simulink model "sldemo_lct_work"  (Simulink 7.6)
settings: Solver=ode5  StartTime=0.0  StopTime=1  RelTol=1e-3
PreLoadFcn:
  | load sldemo_lct_data.mat
Description:
  | Structure Arguments Using Buses
settings Model: Creator=The MathWorks Inc.  ExtModeAutoUpdateStatusClock=off
settings DataIOCC: SignalLoggingName=logsOut
settings OptimizationCC: InlineParams=on  InlineInvariantSignals=on  InitFltsAndDblsToZero=on
settings DebuggingCC: CheckExecutionContextPreStartOutputMsg=on  CheckExecutionContextRuntimeOutputMsg=on  SignalResolutionControl=TryResolveAllWithWarning  SolverPrmCheckMsg=none  MultiTaskDSMMsg=warning  MultiTaskCondExecSysMsg=none  BusObjectLabelMismatch=error  StrictBusMsg=ErrorOnBusTreatedAsVector
settings HardwareCC: TargetHWDeviceType=32-bit Generic
settings ModelReferenceCC: UpdateModelReferenceTargets=IfOutOfDate
settings RTWCC: GenerateReport=on  RetainRTWFile=on  ProcessScript=grt_make_rtw_hook  CustomInclude=.\src  LaunchReport=on  IncludeERTFirstTime=on
settings GRTTargetCC: TargetFcnLib=ansi_tfl_tmw.mat

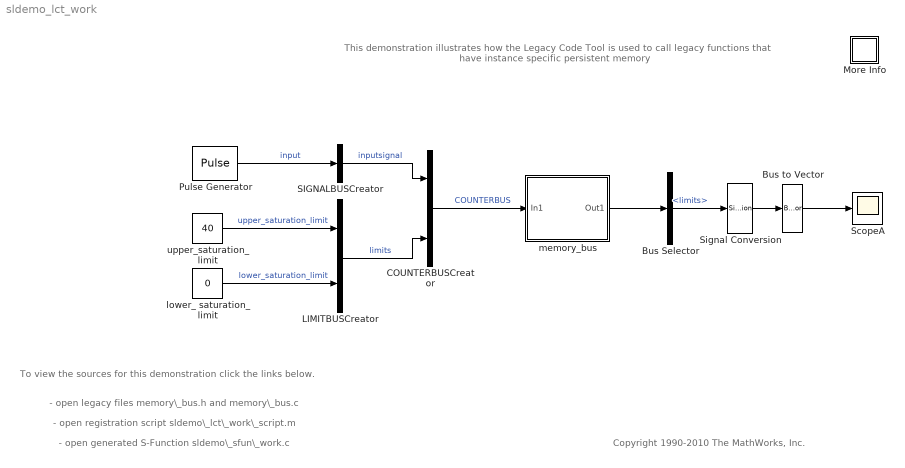
== system sldemo_lct_work ==
  note: This demonstration illustrates how the Legacy Code Tool is used to
      | call legacy functions that have instance specific persistent memory
  note: Copyright 1990-2010 The MathWorks, Inc.
  note: - open legacy files memory\_bus.h and memory\_bus.c
  note: To view the sources for this demonstration
      | click the links below.
  note: - open registration script sldemo\_lct\_work\_script.m
  note: - open generated S-Function sldemo\_sfun\_work.c
  Bus Selector : BusSelector  OutputSignals=limits
  Bus to Vector : BusToVector
  COUNTERBUSCreator : BusCreator  Inputs=2  OutDataTypeStr=Bus: COUNTERBUS  NonVirtualBus=on
  LIMITBUSCreator : BusCreator  Inputs=2  OutDataTypeStr=Bus: LIMITBUS  NonVirtualBus=on
  More Info : Subsystem
      settings: OpenFcn=showdemo('sldemo_lct_work_script')
      mask Display: disp('?')
  Pulse Generator : DiscretePulseGenerator  Amplitude=int32(1)  SampleTime=0.1
  SIGNALBUSCreator : BusCreator  Inputs=1  OutDataTypeStr=Bus: SIGNALBUS  NonVirtualBus=on
  ScopeA : Scope
      settings: TimeRange=1  YMin=-10  YMax=40  SaveName=ScopeDataA  DataFormat=Array
  Signal Conversion : SignalConversion  ConversionOutput=Virtual bus
  lower_ saturation_ limit : Constant  Value=0  OutDataTypeStr=int32
  memory_bus : Subsystem
  upper_saturation_limit : Constant  Value=40  OutDataTypeStr=int32
  wires:
  upper_saturation_limit/1 -> LIMITBUSCreator/1  "upper_saturation_limit"
  lower_ saturation_ limit/1 -> LIMITBUSCreator/2  "lower_saturation_limit"
  LIMITBUSCreator/1 -> COUNTERBUSCreator/2  "limits"
  Pulse Generator/1 -> SIGNALBUSCreator/1  "input"
  SIGNALBUSCreator/1 -> COUNTERBUSCreator/1  "inputsignal"
  memory_bus/1(Out1) -> Bus Selector/1
  COUNTERBUSCreator/1 -> memory_bus/1(In1)  "COUNTERBUS"
  Bus Selector/1 -> Signal Conversion/1  "<limits>"
  Signal Conversion/1 -> Bus to Vector/1
  Bus to Vector/1 -> ScopeA/1

== system sldemo_lct_work/More Info ==

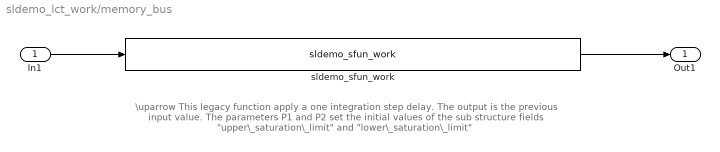
== system sldemo_lct_work/memory_bus ==
  note: \uparrow
      | This legacy function apply a one integration step delay. The output is the previous input value.
      | The parameters P1 and P2 set the initial values of the sub structure fields "upper\_saturation\_limit" and
      | "lower\_saturation\_limit"
  In1 : Inport  OutDataTypeStr=Bus: COUNTERBUS
  sldemo_sfun_work : S-Function  FunctionName=sldemo_sfun_work  Parameters=SParameter1, SParameter2  EnableBusSupport=off  mask(Legacy Function){SFunctionSpec=void memory_bus_step(COUNTERBUS u1[1], COUNTERBUS work1[1], COUNTERBUS y1[1]), SParameter1=10, SParameter2=-10, ShowSpec=on}
      mask prompts: SParameter1 "P1:"; SParameter2 "P2:"; ShowSpec "Display function specification"
      mask help:
      | This block allows you to call the legacy functions specified by the following Legacy Code Tool definition:
      | def.SFunctionName = 'sldemo_sfun_work';
      | def.InitializeConditionsFcnSpec = 'void memory_bus_init(COUNTERBUS work1[1], int32 p1, int32 p2)';
      | def.OutputFcnSpec = 'void memory_bus_step(COUNTERBUS u1[1], COUNTERBUS work1[1], COUNTERBUS y1[1])';
      | def.HeaderFiles = {'memory_bus.h'};
      | def.SourceFiles = {'memory_bus.c'};
      | def.IncPaths = {'sldemo_lct_src'};
      | def.SrcPaths = {'sldemo_lct_src'};
      mask Help: <p>This block was generated automatically by the Legacy Code Tool. For detailed help on this tool, call<a href="matlab:legacy_code('help')"> legacy_code('help')</a>.</p>
      mask CallbackString:
      | |||if strcmp(get_param(gcbh, 'ShowSpec'), 'on')
      |   set_param(gcbh, 'MaskDisplay', sprintf('fprintf(''%s'');', get_param(gcbh, 'SFunctionSpec')));
      | else
      |   set_param(gcbh, 'MaskDisplay', sprintf('fprintf(''%s'');', get_param(gcbh, 'FunctionName')));
      | end
      mask Display: fprintf('void memory_bus_step(COUNTERBUS u1[1], COUNTERBUS work1[1], COUNTERBUS y1[1])');
  Out1 : Outport  OutDataTypeStr=Bus: COUNTERBUS  InitialOutput=0
  wires:
  In1/1 -> sldemo_sfun_work/1
  sldemo_sfun_work/1 -> Out1/1
